simulink subsystem "Sonars"  (R2023b)
settings: Solver=VariableStepAuto  StartTime=0.0  StopTime=10.0  RelTol=1e-3
libraries: arduinolib x2
settings Model: Creator=Carlos  LastModifiedBy=Carlos

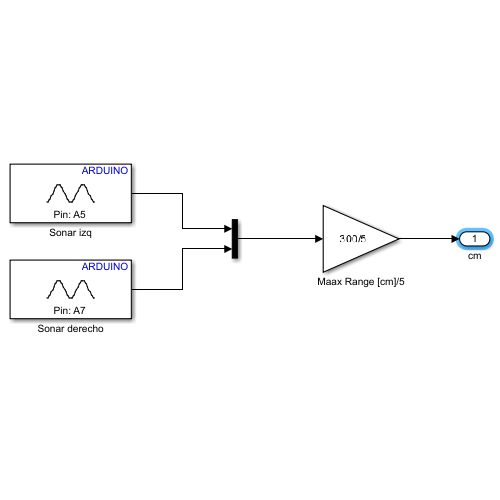
[thumbnail: Simulink's stored preview of the top-level diagram]
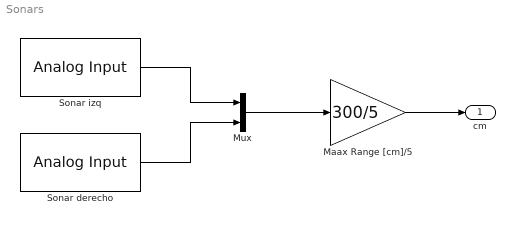
== system Sonars ==
  Maax Range [cm]/5 : Gain  Gain=300/5
  Mux : Mux  Inputs=2
  Sonar derecho : arduinolib/Analog Input  pinNumber=7  ReadResultsOnly=off  ConversionTriggerSource=Software  ExternalTriggerType=uint32( 0 )  OutputDataType=uint16  EnableConversionCompleteNotify=off  EnableOuputStatus=off  SampleTime=.1  blockPlatform=arduino
  Sonar izq : arduinolib/Analog Input  pinNumber=5  ReadResultsOnly=off  ConversionTriggerSource=Software  ExternalTriggerType=uint32( 0 )  OutputDataType=uint16  EnableConversionCompleteNotify=off  EnableOuputStatus=off  SampleTime=.1  blockPlatform=arduino
  cm : Outport
  wires:
  Mux/1 -> Maax Range [cm]/5/1
  Sonar izq/1 -> Mux/1
  Sonar derecho/1 -> Mux/2
  Maax Range [cm]/5/1 -> cm/1
